simulink model "BuildingHeatLoadCalc"  (R2026a)
settings: Solver=ode1be  StopTime=31532400  FixedStep=3600  AbsTol=1e-3
undefined symbols (not defined in the file): BuildingThermalLib, lib_BuildingThermal
libraries: ExternalWall_lib x47, WallSelector_lib x36, fl_lib x32, RoomWithAirVolume x15, nesl_utility x4, TemperatureSource_lib x1, DayScheduler_lib x1, SolarRadiationAtLocation_lib x1
(part 2 of 5)

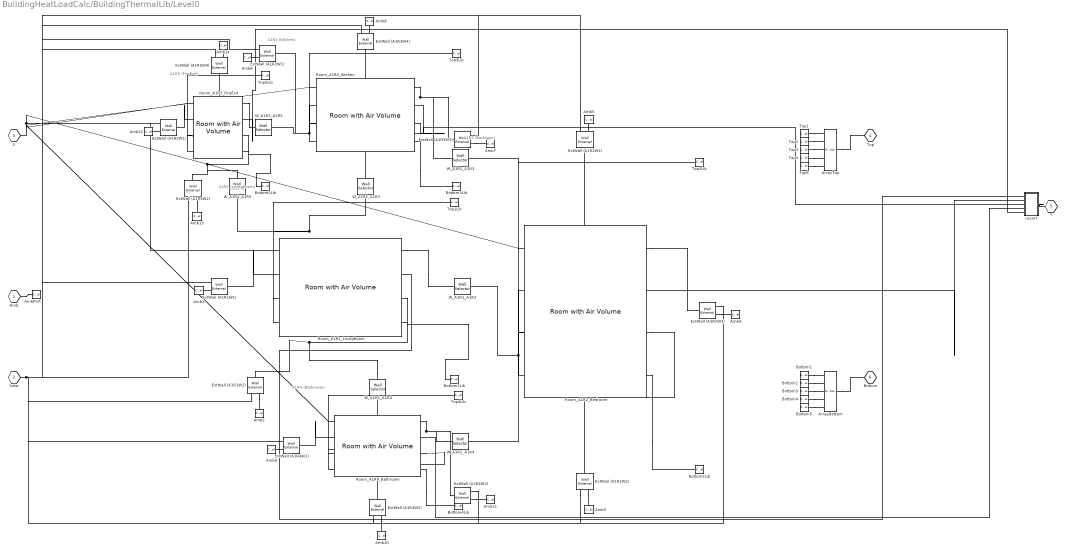
== system BuildingHeatLoadCalc/BuildingThermalLib/Level0 ==
  note: A1R1 (LivingRoom)
  note: A1R2 (Bedroom)
  note: A1R3 (Kitchen)
  note: A1R4 (Bathroom)
  note: A1R5 (FireExit)
  Amb{1..14} (14 alike) : ConnectionLabel  Label=A
  AmbPort : ConnectionLabel  Label=A
  ArrayBottom : SimscapeArrayConnection  Domain=foundation.thermal.thermal  ConcatenateDimension=1  NumScalarElements=5
  ArrayTop : SimscapeArrayConnection  Domain=foundation.thermal.thermal  ConcatenateDimension=1  NumScalarElements=5
  Bottom1 : ConnectionLabel  Label=Bottom1
  Bottom1Lib : ConnectionLabel  Label=Bottom1
  Bottom2 : ConnectionLabel  Label=Bottom2
  Bottom2Lib : ConnectionLabel  Label=Bottom2
  Bottom3 : ConnectionLabel  Label=Bottom3
  Bottom3Lib : ConnectionLabel  Label=Bottom3
  Bottom4 : ConnectionLabel  Label=Bottom4
  Bottom4Lib : ConnectionLabel  Label=Bottom4
  Bottom5 : ConnectionLabel  Label=Bottom5
  Bottom5Lib : ConnectionLabel  Label=Bottom5
  ExtWall (A1R1W1) : ExternalWall_lib/Wall External  extWallModel=wallExternalModelOption.wallSolarWin  wallLength=2.4384 % Parameterized on : 09-Jun-2026 19:35:12 m  wallHeight=3.048 % Parameterized on : 09-Jun-2026 19:35:12 m  wallThickness=0.07 % Parameterized on : 09-Jun-2026 19:35:12 m  wallMaterialDen=2000 % Parameterized on : 09-Jun-2026 19:35:13 kg/m^3  wallMaterialCp=1100 % Parameterized on : 09-Jun-2026 19:35:13 J/(K*kg)  wallAbsorptivity=0.6 % Parameterized on : 09-Jun-2026 19:35:13  wallThermalK=1.4 % Parameterized on : 09-Jun-2026 19:35:13 W/(K*m)  winLength=2.0401 % Parameterized on : 09-Jun-2026 19:35:12 m  winHeight=2.5501 % Parameterized on : 09-Jun-2026 19:35:12 m  winThickness=0.005 % Parameterized on : 09-Jun-2026 19:35:13 m  winMaterialDen=4000 % Parameterized on : 09-Jun-2026 19:35:13 kg/m^3  winMaterialCp=840 % Parameterized on : 09-Jun-2026 19:35:13 J/(K*kg)  winAbsorptivity=0.4 % Parameterized on : 09-Jun-2026 19:35:13  winThermalK=1 % Parameterized on : 09-Jun-2026 19:35:13 W/(K*m)  winTransmissivity=0.2 % Parameterized on : 09-Jun-2026 19:35:13  ventLength=0.1 m  ventHeight=0.1 m  extToWallHTC=20 % Parameterized on : 09-Jun-2026 19:35:13 W/(K*m^2)  intToRoomHTC=30 % Parameterized on : 09-Jun-2026 19:35:13 W/(K*m^2)  iniT=275.8 % Parameterized on : 09-Jun-2026 19:38:28 K  latitude=47.376 % Parameterized on : 09-Jun-2026 19:38:29  longitude=8.541 % Parameterized on : 09-Jun-2026 19:38:29  localTime=15.00 % Parameterized on : 09-Jun-2026 19:38:29  dayLightS=0 % Parameterized on : 09-Jun-2026 19:38:29  surfAngle=90 % Parameterized on : 09-Jun-2026 19:35:12 deg  surfUnitV="[-0.96593    -0.25882] % Parameterized on : 09-Jun-2026 19:35:12"  startYear=2024 % Parameterized on : 09-Jun-2026 19:38:29  startMonth=1 % Parameterized on : 09-Jun-2026 19:38:29  startDay=1 % Parameterized on : 09-Jun-2026 19:38:29  startHr=1 % Parameterized on : 09-Jun-2026 19:38:29  numHrsData=8760 % Parameterized on : 09-Jun-2026 19:38:29  interp_method=simscape.enum.interpolation.linear  extrap_method=simscape.enum.extrapolation.nearest
  ExtWall (A1R1W2) : ExternalWall_lib/Wall External  extWallModel=wallExternalModelOption.wallSolarWin  wallLength=3.048 % Parameterized on : 09-Jun-2026 19:35:12 m  wallHeight=3.048 % Parameterized on : 09-Jun-2026 19:35:12 m  wallThickness=0.07 % Parameterized on : 09-Jun-2026 19:35:12 m  wallMaterialDen=2000 % Parameterized on : 09-Jun-2026 19:35:13 kg/m^3  wallMaterialCp=1100 % Parameterized on : 09-Jun-2026 19:35:13 J/(K*kg)  wallAbsorptivity=0.6 % Parameterized on : 09-Jun-2026 19:35:13  wallThermalK=1.4 % Parameterized on : 09-Jun-2026 19:35:13 W/(K*m)  winLength=2.1552 % Parameterized on : 09-Jun-2026 19:35:12 m  winHeight=2.1553 % Parameterized on : 09-Jun-2026 19:35:12 m  winThickness=0.005 % Parameterized on : 09-Jun-2026 19:35:13 m  winMaterialDen=4000 % Parameterized on : 09-Jun-2026 19:35:13 kg/m^3  winMaterialCp=840 % Parameterized on : 09-Jun-2026 19:35:13 J/(K*kg)  winAbsorptivity=0.4 % Parameterized on : 09-Jun-2026 19:35:13  winThermalK=1 % Parameterized on : 09-Jun-2026 19:35:13 W/(K*m)  winTransmissivity=0.2 % Parameterized on : 09-Jun-2026 19:35:13  ventLength=0.1 m  ventHeight=0.1 m  extToWallHTC=20 % Parameterized on : 09-Jun-2026 19:35:13 W/(K*m^2)  intToRoomHTC=30 % Parameterized on : 09-Jun-2026 19:35:13 W/(K*m^2)  iniT=275.8 % Parameterized on : 09-Jun-2026 19:38:28 K  latitude=47.376 % Parameterized on : 09-Jun-2026 19:38:29  longitude=8.541 % Parameterized on : 09-Jun-2026 19:38:29  localTime=15.00 % Parameterized on : 09-Jun-2026 19:38:29  dayLightS=0 % Parameterized on : 09-Jun-2026 19:38:29  surfAngle=90 % Parameterized on : 09-Jun-2026 19:35:12 deg  surfUnitV="[-0.25882     0.96593] % Parameterized on : 09-Jun-2026 19:35:12"  startYear=2024 % Parameterized on : 09-Jun-2026 19:38:29  startMonth=1 % Parameterized on : 09-Jun-2026 19:38:29  startDay=1 % Parameterized on : 09-Jun-2026 19:38:29  startHr=1 % Parameterized on : 09-Jun-2026 19:38:29  numHrsData=8760 % Parameterized on : 09-Jun-2026 19:38:29  interp_method=simscape.enum.interpolation.linear  extrap_method=simscape.enum.extrapolation.nearest
  ExtWall (A1R2W2) : ExternalWall_lib/Wall External  extWallModel=wallExternalModelOption.wallSolar  wallLength=3.048 % Parameterized on : 09-Jun-2026 19:35:12 m  wallHeight=3.048 % Parameterized on : 09-Jun-2026 19:35:12 m  wallThickness=0.07 % Parameterized on : 09-Jun-2026 19:35:12 m  wallMaterialDen=2000 % Parameterized on : 09-Jun-2026 19:35:13 kg/m^3  wallMaterialCp=1100 % Parameterized on : 09-Jun-2026 19:35:13 J/(K*kg)  wallAbsorptivity=0.6 % Parameterized on : 09-Jun-2026 19:35:13  wallThermalK=1.4 % Parameterized on : 09-Jun-2026 19:35:13 W/(K*m)  winLength=1 m  winHeight=0.5 m  winThickness=0.007 m  winMaterialDen=2500 kg/m^3  winMaterialCp=787 J/(K*kg)  winAbsorptivity=0.35  winThermalK=1 W/(K*m)  winTransmissivity=0.45  ventLength=0.1 m  ventHeight=0.1 m  extToWallHTC=20 % Parameterized on : 09-Jun-2026 19:35:13 W/(K*m^2)  intToRoomHTC=30 % Parameterized on : 09-Jun-2026 19:35:13 W/(K*m^2)  iniT=275.8 % Parameterized on : 09-Jun-2026 19:38:28 K  latitude=47.376 % Parameterized on : 09-Jun-2026 19:38:29  longitude=8.541 % Parameterized on : 09-Jun-2026 19:38:29  localTime=15.00 % Parameterized on : 09-Jun-2026 19:38:29  dayLightS=0 % Parameterized on : 09-Jun-2026 19:38:29  surfAngle=90 % Parameterized on : 09-Jun-2026 19:35:12 deg  surfUnitV="[-0.25882     0.96593] % Parameterized on : 09-Jun-2026 19:35:12"  startYear=2024 % Parameterized on : 09-Jun-2026 19:38:29  startMonth=1 % Parameterized on : 09-Jun-2026 19:38:29  startDay=1 % Parameterized on : 09-Jun-2026 19:38:29  startHr=1 % Parameterized on : 09-Jun-2026 19:38:29  numHrsData=8760 % Parameterized on : 09-Jun-2026 19:38:29  interp_method=simscape.enum.interpolation.linear  extrap_method=simscape.enum.extrapolation.nearest
  ExtWall (A1R2W3) : ExternalWall_lib/Wall External  extWallModel=wallExternalModelOption.wallSolarWin  wallLength=4.2672 % Parameterized on : 09-Jun-2026 19:35:12 m  wallHeight=3.048 % Parameterized on : 09-Jun-2026 19:35:12 m  wallThickness=0.07 % Parameterized on : 09-Jun-2026 19:35:12 m  wallMaterialDen=2000 % Parameterized on : 09-Jun-2026 19:35:13 kg/m^3  wallMaterialCp=1100 % Parameterized on : 09-Jun-2026 19:35:13 J/(K*kg)  wallAbsorptivity=0.6 % Parameterized on : 09-Jun-2026 19:35:13  wallThermalK=1.4 % Parameterized on : 09-Jun-2026 19:35:13 W/(K*m)  winLength=3.5702 % Parameterized on : 09-Jun-2026 19:35:12 m  winHeight=2.5501 % Parameterized on : 09-Jun-2026 19:35:12 m  winThickness=0.005 % Parameterized on : 09-Jun-2026 19:35:13 m  winMaterialDen=4000 % Parameterized on : 09-Jun-2026 19:35:13 kg/m^3  winMaterialCp=840 % Parameterized on : 09-Jun-2026 19:35:13 J/(K*kg)  winAbsorptivity=0.4 % Parameterized on : 09-Jun-2026 19:35:13  winThermalK=1 % Parameterized on : 09-Jun-2026 19:35:13 W/(K*m)  winTransmissivity=0.2 % Parameterized on : 09-Jun-2026 19:35:13  ventLength=0.1 m  ventHeight=0.1 m  extToWallHTC=20 % Parameterized on : 09-Jun-2026 19:35:13 W/(K*m^2)  intToRoomHTC=30 % Parameterized on : 09-Jun-2026 19:35:13 W/(K*m^2)  iniT=275.8 % Parameterized on : 09-Jun-2026 19:38:28 K  latitude=47.376 % Parameterized on : 09-Jun-2026 19:38:29  longitude=8.541 % Parameterized on : 09-Jun-2026 19:38:29  localTime=15.00 % Parameterized on : 09-Jun-2026 19:38:29  dayLightS=0 % Parameterized on : 09-Jun-2026 19:38:29  surfAngle=90 % Parameterized on : 09-Jun-2026 19:35:12 deg  surfUnitV="[0.96593     0.25882] % Parameterized on : 09-Jun-2026 19:35:12"  startYear=2024 % Parameterized on : 09-Jun-2026 19:38:29  startMonth=1 % Parameterized on : 09-Jun-2026 19:38:29  startDay=1 % Parameterized on : 09-Jun-2026 19:38:29  startHr=1 % Parameterized on : 09-Jun-2026 19:38:29  numHrsData=8760 % Parameterized on : 09-Jun-2026 19:38:29  interp_method=simscape.enum.interpolation.linear  extrap_method=simscape.enum.extrapolation.nearest
  ExtWall (A1R2W4) : ExternalWall_lib/Wall External  extWallModel=wallExternalModelOption.wallSolarWin  wallLength=3.048 % Parameterized on : 09-Jun-2026 19:35:12 m  wallHeight=3.048 % Parameterized on : 09-Jun-2026 19:35:12 m  wallThickness=0.07 % Parameterized on : 09-Jun-2026 19:35:12 m  wallMaterialDen=2000 % Parameterized on : 09-Jun-2026 19:35:13 kg/m^3  wallMaterialCp=1100 % Parameterized on : 09-Jun-2026 19:35:13 J/(K*kg)  wallAbsorptivity=0.6 % Parameterized on : 09-Jun-2026 19:35:13  wallThermalK=1.4 % Parameterized on : 09-Jun-2026 19:35:13 W/(K*m)  winLength=2.1552 % Parameterized on : 09-Jun-2026 19:35:12 m  winHeight=2.1553 % Parameterized on : 09-Jun-2026 19:35:12 m  winThickness=0.005 % Parameterized on : 09-Jun-2026 19:35:13 m  winMaterialDen=4000 % Parameterized on : 09-Jun-2026 19:35:13 kg/m^3  winMaterialCp=840 % Parameterized on : 09-Jun-2026 19:35:13 J/(K*kg)  winAbsorptivity=0.4 % Parameterized on : 09-Jun-2026 19:35:13  winThermalK=1 % Parameterized on : 09-Jun-2026 19:35:13 W/(K*m)  winTransmissivity=0.2 % Parameterized on : 09-Jun-2026 19:35:13  ventLength=0.1 m  ventHeight=0.1 m  extToWallHTC=20 % Parameterized on : 09-Jun-2026 19:35:13 W/(K*m^2)  intToRoomHTC=30 % Parameterized on : 09-Jun-2026 19:35:13 W/(K*m^2)  iniT=275.8 % Parameterized on : 09-Jun-2026 19:38:28 K  latitude=47.376 % Parameterized on : 09-Jun-2026 19:38:29  longitude=8.541 % Parameterized on : 09-Jun-2026 19:38:29  localTime=15.00 % Parameterized on : 09-Jun-2026 19:38:29  dayLightS=0 % Parameterized on : 09-Jun-2026 19:38:29  surfAngle=90 % Parameterized on : 09-Jun-2026 19:35:12 deg  surfUnitV="[0.25882    -0.96593] % Parameterized on : 09-Jun-2026 19:35:12"  startYear=2024 % Parameterized on : 09-Jun-2026 19:38:29  startMonth=1 % Parameterized on : 09-Jun-2026 19:38:29  startDay=1 % Parameterized on : 09-Jun-2026 19:38:29  startHr=1 % Parameterized on : 09-Jun-2026 19:38:29  numHrsData=8760 % Parameterized on : 09-Jun-2026 19:38:29  interp_method=simscape.enum.interpolation.linear  extrap_method=simscape.enum.extrapolation.nearest
  ExtWall (A1R3W1) : ExternalWall_lib/Wall External  extWallModel=wallExternalModelOption.wallSolar  wallLength=1.8288 % Parameterized on : 09-Jun-2026 19:35:12 m  wallHeight=3.048 % Parameterized on : 09-Jun-2026 19:35:12 m  wallThickness=0.07 % Parameterized on : 09-Jun-2026 19:35:12 m  wallMaterialDen=2000 % Parameterized on : 09-Jun-2026 19:35:13 kg/m^3  wallMaterialCp=1100 % Parameterized on : 09-Jun-2026 19:35:13 J/(K*kg)  wallAbsorptivity=0.6 % Parameterized on : 09-Jun-2026 19:35:13  wallThermalK=1.4 % Parameterized on : 09-Jun-2026 19:35:13 W/(K*m)  winLength=1 m  winHeight=0.5 m  winThickness=0.007 m  winMaterialDen=2500 kg/m^3  winMaterialCp=787 J/(K*kg)  winAbsorptivity=0.35  winThermalK=1 W/(K*m)  winTransmissivity=0.45  ventLength=0.1 m  ventHeight=0.1 m  extToWallHTC=20 % Parameterized on : 09-Jun-2026 19:35:13 W/(K*m^2)  intToRoomHTC=30 % Parameterized on : 09-Jun-2026 19:35:13 W/(K*m^2)  iniT=275.8 % Parameterized on : 09-Jun-2026 19:38:28 K  latitude=47.376 % Parameterized on : 09-Jun-2026 19:38:29  longitude=8.541 % Parameterized on : 09-Jun-2026 19:38:29  localTime=15.00 % Parameterized on : 09-Jun-2026 19:38:29  dayLightS=0 % Parameterized on : 09-Jun-2026 19:38:29  surfAngle=90 % Parameterized on : 09-Jun-2026 19:35:12 deg  surfUnitV="[-0.96593    -0.25882] % Parameterized on : 09-Jun-2026 19:35:12"  startYear=2024 % Parameterized on : 09-Jun-2026 19:38:29  startMonth=1 % Parameterized on : 09-Jun-2026 19:38:29  startDay=1 % Parameterized on : 09-Jun-2026 19:38:29  startHr=1 % Parameterized on : 09-Jun-2026 19:38:29  numHrsData=8760 % Parameterized on : 09-Jun-2026 19:38:29  interp_method=simscape.enum.interpolation.linear  extrap_method=simscape.enum.extrapolation.nearest
  ExtWall (A1R3W3) : ExternalWall_lib/Wall External  extWallModel=wallExternalModelOption.wallSolarWin  wallLength=1.8289 % Parameterized on : 09-Jun-2026 19:35:12 m  wallHeight=3.048 % Parameterized on : 09-Jun-2026 19:35:12 m  wallThickness=0.07 % Parameterized on : 09-Jun-2026 19:35:12 m  wallMaterialDen=2000 % Parameterized on : 09-Jun-2026 19:35:13 kg/m^3  wallMaterialCp=1100 % Parameterized on : 09-Jun-2026 19:35:13 J/(K*kg)  wallAbsorptivity=0.6 % Parameterized on : 09-Jun-2026 19:35:13  wallThermalK=1.4 % Parameterized on : 09-Jun-2026 19:35:13 W/(K*m)  winLength=1.5301 % Parameterized on : 09-Jun-2026 19:35:12 m  winHeight=2.5501 % Parameterized on : 09-Jun-2026 19:35:12 m  winThickness=0.005 % Parameterized on : 09-Jun-2026 19:35:13 m  winMaterialDen=4000 % Parameterized on : 09-Jun-2026 19:35:13 kg/m^3  winMaterialCp=840 % Parameterized on : 09-Jun-2026 19:35:13 J/(K*kg)  winAbsorptivity=0.4 % Parameterized on : 09-Jun-2026 19:35:13  winThermalK=1 % Parameterized on : 09-Jun-2026 19:35:13 W/(K*m)  winTransmissivity=0.2 % Parameterized on : 09-Jun-2026 19:35:13  ventLength=0.1 m  ventHeight=0.1 m  extToWallHTC=20 % Parameterized on : 09-Jun-2026 19:35:13 W/(K*m^2)  intToRoomHTC=30 % Parameterized on : 09-Jun-2026 19:35:13 W/(K*m^2)  iniT=275.8 % Parameterized on : 09-Jun-2026 19:38:28 K  latitude=47.376 % Parameterized on : 09-Jun-2026 19:38:29  longitude=8.541 % Parameterized on : 09-Jun-2026 19:38:29  localTime=15.00 % Parameterized on : 09-Jun-2026 19:38:29  dayLightS=0 % Parameterized on : 09-Jun-2026 19:38:29  surfAngle=90 % Parameterized on : 09-Jun-2026 19:35:12 deg  surfUnitV="[0.96593     0.25882] % Parameterized on : 09-Jun-2026 19:35:12"  startYear=2024 % Parameterized on : 09-Jun-2026 19:38:29  startMonth=1 % Parameterized on : 09-Jun-2026 19:38:29  startDay=1 % Parameterized on : 09-Jun-2026 19:38:29  startHr=1 % Parameterized on : 09-Jun-2026 19:38:29  numHrsData=8760 % Parameterized on : 09-Jun-2026 19:38:29  interp_method=simscape.enum.interpolation.linear  extrap_method=simscape.enum.extrapolation.nearest
  ExtWall (A1R3W4) : ExternalWall_lib/Wall External  extWallModel=wallExternalModelOption.wallSolarWin  wallLength=2.4385 % Parameterized on : 09-Jun-2026 19:35:12 m  wallHeight=3.048 % Parameterized on : 09-Jun-2026 19:35:12 m  wallThickness=0.07 % Parameterized on : 09-Jun-2026 19:35:12 m  wallMaterialDen=2000 % Parameterized on : 09-Jun-2026 19:35:13 kg/m^3  wallMaterialCp=1100 % Parameterized on : 09-Jun-2026 19:35:13 J/(K*kg)  wallAbsorptivity=0.6 % Parameterized on : 09-Jun-2026 19:35:13  wallThermalK=1.4 % Parameterized on : 09-Jun-2026 19:35:13 W/(K*m)  winLength=2.0402 % Parameterized on : 09-Jun-2026 19:35:12 m  winHeight=2.5501 % Parameterized on : 09-Jun-2026 19:35:12 m  winThickness=0.005 % Parameterized on : 09-Jun-2026 19:35:13 m  winMaterialDen=4000 % Parameterized on : 09-Jun-2026 19:35:13 kg/m^3  winMaterialCp=840 % Parameterized on : 09-Jun-2026 19:35:13 J/(K*kg)  winAbsorptivity=0.4 % Parameterized on : 09-Jun-2026 19:35:13  winThermalK=1 % Parameterized on : 09-Jun-2026 19:35:13 W/(K*m)  winTransmissivity=0.2 % Parameterized on : 09-Jun-2026 19:35:13  ventLength=0.1 m  ventHeight=0.1 m  extToWallHTC=20 % Parameterized on : 09-Jun-2026 19:35:13 W/(K*m^2)  intToRoomHTC=30 % Parameterized on : 09-Jun-2026 19:35:13 W/(K*m^2)  iniT=275.8 % Parameterized on : 09-Jun-2026 19:38:28 K  latitude=47.376 % Parameterized on : 09-Jun-2026 19:38:29  longitude=8.541 % Parameterized on : 09-Jun-2026 19:38:29  localTime=15.00 % Parameterized on : 09-Jun-2026 19:38:29  dayLightS=0 % Parameterized on : 09-Jun-2026 19:38:29  surfAngle=90 % Parameterized on : 09-Jun-2026 19:35:12 deg  surfUnitV="[0.25882    -0.96593] % Parameterized on : 09-Jun-2026 19:35:12"  startYear=2024 % Parameterized on : 09-Jun-2026 19:38:29  startMonth=1 % Parameterized on : 09-Jun-2026 19:38:29  startDay=1 % Parameterized on : 09-Jun-2026 19:38:29  startHr=1 % Parameterized on : 09-Jun-2026 19:38:29  numHrsData=8760 % Parameterized on : 09-Jun-2026 19:38:29  interp_method=simscape.enum.interpolation.linear  extrap_method=simscape.enum.extrapolation.nearest
  ExtWall (A1R4W1) : ExternalWall_lib/Wall External  extWallModel=wallExternalModelOption.wallSolar  wallLength=1.524 % Parameterized on : 09-Jun-2026 19:35:12 m  wallHeight=3.048 % Parameterized on : 09-Jun-2026 19:35:12 m  wallThickness=0.07 % Parameterized on : 09-Jun-2026 19:35:12 m  wallMaterialDen=2000 % Parameterized on : 09-Jun-2026 19:35:13 kg/m^3  wallMaterialCp=1100 % Parameterized on : 09-Jun-2026 19:35:13 J/(K*kg)  wallAbsorptivity=0.6 % Parameterized on : 09-Jun-2026 19:35:13  wallThermalK=1.4 % Parameterized on : 09-Jun-2026 19:35:13 W/(K*m)  winLength=1 m  winHeight=0.5 m  winThickness=0.007 m  winMaterialDen=2500 kg/m^3  winMaterialCp=787 J/(K*kg)  winAbsorptivity=0.35  winThermalK=1 W/(K*m)  winTransmissivity=0.45  ventLength=0.1 m  ventHeight=0.1 m  extToWallHTC=20 % Parameterized on : 09-Jun-2026 19:35:13 W/(K*m^2)  intToRoomHTC=30 % Parameterized on : 09-Jun-2026 19:35:13 W/(K*m^2)  iniT=275.8 % Parameterized on : 09-Jun-2026 19:38:28 K  latitude=47.376 % Parameterized on : 09-Jun-2026 19:38:29  longitude=8.541 % Parameterized on : 09-Jun-2026 19:38:29  localTime=15.00 % Parameterized on : 09-Jun-2026 19:38:29  dayLightS=0 % Parameterized on : 09-Jun-2026 19:38:29  surfAngle=90 % Parameterized on : 09-Jun-2026 19:35:12 deg  surfUnitV="[-0.96593    -0.25882] % Parameterized on : 09-Jun-2026 19:35:12"  startYear=2024 % Parameterized on : 09-Jun-2026 19:38:29  startMonth=1 % Parameterized on : 09-Jun-2026 19:38:29  startDay=1 % Parameterized on : 09-Jun-2026 19:38:29  startHr=1 % Parameterized on : 09-Jun-2026 19:38:29  numHrsData=8760 % Parameterized on : 09-Jun-2026 19:38:29  interp_method=simscape.enum.interpolation.linear  extrap_method=simscape.enum.extrapolation.nearest
  ExtWall (A1R4W2) : ExternalWall_lib/Wall External  extWallModel=wallExternalModelOption.wallSolarWin  wallLength=2.1336 % Parameterized on : 09-Jun-2026 19:35:12 m  wallHeight=3.048 % Parameterized on : 09-Jun-2026 19:35:12 m  wallThickness=0.07 % Parameterized on : 09-Jun-2026 19:35:12 m  wallMaterialDen=2000 % Parameterized on : 09-Jun-2026 19:35:13 kg/m^3  wallMaterialCp=1100 % Parameterized on : 09-Jun-2026 19:35:14 J/(K*kg)  wallAbsorptivity=0.6 % Parameterized on : 09-Jun-2026 19:35:14  wallThermalK=1.4 % Parameterized on : 09-Jun-2026 19:35:14 W/(K*m)  winLength=1.1686 % Parameterized on : 09-Jun-2026 19:35:12 m  winHeight=1.6695 % Parameterized on : 09-Jun-2026 19:35:12 m  winThickness=0.005 % Parameterized on : 09-Jun-2026 19:35:14 m  winMaterialDen=4000 % Parameterized on : 09-Jun-2026 19:35:14 kg/m^3  winMaterialCp=840 % Parameterized on : 09-Jun-2026 19:35:14 J/(K*kg)  winAbsorptivity=0.4 % Parameterized on : 09-Jun-2026 19:35:14  winThermalK=1 % Parameterized on : 09-Jun-2026 19:35:14 W/(K*m)  winTransmissivity=0.2 % Parameterized on : 09-Jun-2026 19:35:14  ventLength=0.1 m  ventHeight=0.1 m  extToWallHTC=20 % Parameterized on : 09-Jun-2026 19:35:14 W/(K*m^2)  intToRoomHTC=30 % Parameterized on : 09-Jun-2026 19:35:14 W/(K*m^2)  iniT=275.8 % Parameterized on : 09-Jun-2026 19:38:28 K  latitude=47.376 % Parameterized on : 09-Jun-2026 19:38:29  longitude=8.541 % Parameterized on : 09-Jun-2026 19:38:29  localTime=15.00 % Parameterized on : 09-Jun-2026 19:38:29  dayLightS=0 % Parameterized on : 09-Jun-2026 19:38:29  surfAngle=90 % Parameterized on : 09-Jun-2026 19:35:12 deg  surfUnitV="[-0.25882     0.96593] % Parameterized on : 09-Jun-2026 19:35:12"  startYear=2024 % Parameterized on : 09-Jun-2026 19:38:29  startMonth=1 % Parameterized on : 09-Jun-2026 19:38:29  startDay=1 % Parameterized on : 09-Jun-2026 19:38:29  startHr=1 % Parameterized on : 09-Jun-2026 19:38:29  numHrsData=8760 % Parameterized on : 09-Jun-2026 19:38:29  interp_method=simscape.enum.interpolation.linear  extrap_method=simscape.enum.extrapolation.nearest
  ExtWall (A1R4W3) : ExternalWall_lib/Wall External  extWallModel=wallExternalModelOption.wallSolar  wallLength=1.524 % Parameterized on : 09-Jun-2026 19:35:12 m  wallHeight=3.048 % Parameterized on : 09-Jun-2026 19:35:12 m  wallThickness=0.07 % Parameterized on : 09-Jun-2026 19:35:12 m  wallMaterialDen=2000 % Parameterized on : 09-Jun-2026 19:35:14 kg/m^3  wallMaterialCp=1100 % Parameterized on : 09-Jun-2026 19:35:14 J/(K*kg)  wallAbsorptivity=0.6 % Parameterized on : 09-Jun-2026 19:35:14  wallThermalK=1.4 % Parameterized on : 09-Jun-2026 19:35:14 W/(K*m)  winLength=1 m  winHeight=0.5 m  winThickness=0.007 m  winMaterialDen=2500 kg/m^3  winMaterialCp=787 J/(K*kg)  winAbsorptivity=0.35  winThermalK=1 W/(K*m)  winTransmissivity=0.45  ventLength=0.1 m  ventHeight=0.1 m  extToWallHTC=20 % Parameterized on : 09-Jun-2026 19:35:14 W/(K*m^2)  intToRoomHTC=30 % Parameterized on : 09-Jun-2026 19:35:14 W/(K*m^2)  iniT=275.8 % Parameterized on : 09-Jun-2026 19:38:28 K  latitude=47.376 % Parameterized on : 09-Jun-2026 19:38:29  longitude=8.541 % Parameterized on : 09-Jun-2026 19:38:29  localTime=15.00 % Parameterized on : 09-Jun-2026 19:38:29  dayLightS=0 % Parameterized on : 09-Jun-2026 19:38:29  surfAngle=90 % Parameterized on : 09-Jun-2026 19:35:12 deg  surfUnitV="[0.96593     0.25882] % Parameterized on : 09-Jun-2026 19:35:12"  startYear=2024 % Parameterized on : 09-Jun-2026 19:38:29  startMonth=1 % Parameterized on : 09-Jun-2026 19:38:29  startDay=1 % Parameterized on : 09-Jun-2026 19:38:29  startHr=1 % Parameterized on : 09-Jun-2026 19:38:29  numHrsData=8760 % Parameterized on : 09-Jun-2026 19:38:29  interp_method=simscape.enum.interpolation.linear  extrap_method=simscape.enum.extrapolation.nearest
  ExtWall (A1R5W1) : ExternalWall_lib/Wall External  extWallModel=wallExternalModelOption.wallSolar  wallLength=1.524 % Parameterized on : 09-Jun-2026 19:35:12 m  wallHeight=3.048 % Parameterized on : 09-Jun-2026 19:35:12 m  wallThickness=0.07 % Parameterized on : 09-Jun-2026 19:35:12 m  wallMaterialDen=2000 % Parameterized on : 09-Jun-2026 19:35:14 kg/m^3  wallMaterialCp=1100 % Parameterized on : 09-Jun-2026 19:35:14 J/(K*kg)  wallAbsorptivity=0.6 % Parameterized on : 09-Jun-2026 19:35:14  wallThermalK=1.4 % Parameterized on : 09-Jun-2026 19:35:14 W/(K*m)  winLength=1 m  winHeight=0.5 m  winThickness=0.007 m  winMaterialDen=2500 kg/m^3  winMaterialCp=787 J/(K*kg)  winAbsorptivity=0.35  winThermalK=1 W/(K*m)  winTransmissivity=0.45  ventLength=0.1 m  ventHeight=0.1 m  extToWallHTC=20 % Parameterized on : 09-Jun-2026 19:35:14 W/(K*m^2)  intToRoomHTC=30 % Parameterized on : 09-Jun-2026 19:35:14 W/(K*m^2)  iniT=275.8 % Parameterized on : 09-Jun-2026 19:38:28 K  latitude=47.376 % Parameterized on : 09-Jun-2026 19:38:29  longitude=8.541 % Parameterized on : 09-Jun-2026 19:38:29  localTime=15.00 % Parameterized on : 09-Jun-2026 19:38:29  dayLightS=0 % Parameterized on : 09-Jun-2026 19:38:29  surfAngle=90 % Parameterized on : 09-Jun-2026 19:35:12 deg  surfUnitV="[-0.96593    -0.25882] % Parameterized on : 09-Jun-2026 19:35:12"  startYear=2024 % Parameterized on : 09-Jun-2026 19:38:29  startMonth=1 % Parameterized on : 09-Jun-2026 19:38:29  startDay=1 % Parameterized on : 09-Jun-2026 19:38:29  startHr=1 % Parameterized on : 09-Jun-2026 19:38:29  numHrsData=8760 % Parameterized on : 09-Jun-2026 19:38:29  interp_method=simscape.enum.interpolation.linear  extrap_method=simscape.enum.extrapolation.nearest
  ExtWall (A1R5W2) : ExternalWall_lib/Wall External  extWallModel=wallExternalModelOption.wallSolar  wallLength=1.2192 % Parameterized on : 09-Jun-2026 19:35:12 m  wallHeight=3.048 % Parameterized on : 09-Jun-2026 19:35:12 m  wallThickness=0.07 % Parameterized on : 09-Jun-2026 19:35:12 m  wallMaterialDen=2000 % Parameterized on : 09-Jun-2026 19:35:14 kg/m^3  wallMaterialCp=1100 % Parameterized on : 09-Jun-2026 19:35:14 J/(K*kg)  wallAbsorptivity=0.6 % Parameterized on : 09-Jun-2026 19:35:14  wallThermalK=1.4 % Parameterized on : 09-Jun-2026 19:35:14 W/(K*m)  winLength=1 m  winHeight=0.5 m  winThickness=0.007 m  winMaterialDen=2500 kg/m^3  winMaterialCp=787 J/(K*kg)  winAbsorptivity=0.35  winThermalK=1 W/(K*m)  winTransmissivity=0.45  ventLength=0.1 m  ventHeight=0.1 m  extToWallHTC=20 % Parameterized on : 09-Jun-2026 19:35:14 W/(K*m^2)  intToRoomHTC=30 % Parameterized on : 09-Jun-2026 19:35:14 W/(K*m^2)  iniT=275.8 % Parameterized on : 09-Jun-2026 19:38:28 K  latitude=47.376 % Parameterized on : 09-Jun-2026 19:38:29  longitude=8.541 % Parameterized on : 09-Jun-2026 19:38:29  localTime=15.00 % Parameterized on : 09-Jun-2026 19:38:29  dayLightS=0 % Parameterized on : 09-Jun-2026 19:38:29  surfAngle=90 % Parameterized on : 09-Jun-2026 19:35:12 deg  surfUnitV="[-0.25882     0.96593] % Parameterized on : 09-Jun-2026 19:35:12"  startYear=2024 % Parameterized on : 09-Jun-2026 19:38:29  startMonth=1 % Parameterized on : 09-Jun-2026 19:38:29  startDay=1 % Parameterized on : 09-Jun-2026 19:38:29  startHr=1 % Parameterized on : 09-Jun-2026 19:38:29  numHrsData=8760 % Parameterized on : 09-Jun-2026 19:38:29  interp_method=simscape.enum.interpolation.linear  extrap_method=simscape.enum.extrapolation.nearest
  ExtWall (A1R5W4) : ExternalWall_lib/Wall External  extWallModel=wallExternalModelOption.wallSolarWin  wallLength=1.2192 % Parameterized on : 09-Jun-2026 19:35:12 m  wallHeight=3.048 % Parameterized on : 09-Jun-2026 19:35:12 m  wallThickness=0.07 % Parameterized on : 09-Jun-2026 19:35:12 m  wallMaterialDen=2000 % Parameterized on : 09-Jun-2026 19:35:14 kg/m^3  wallMaterialCp=1100 % Parameterized on : 09-Jun-2026 19:35:14 J/(K*kg)  wallAbsorptivity=0.6 % Parameterized on : 09-Jun-2026 19:35:14  wallThermalK=1.4 % Parameterized on : 09-Jun-2026 19:35:14 W/(K*m)  winLength=0.9444 % Parameterized on : 09-Jun-2026 19:35:12 m  winHeight=2.361 % Parameterized on : 09-Jun-2026 19:35:12 m  winThickness=0.005 % Parameterized on : 09-Jun-2026 19:35:14 m  winMaterialDen=4000 % Parameterized on : 09-Jun-2026 19:35:14 kg/m^3  winMaterialCp=840 % Parameterized on : 09-Jun-2026 19:35:14 J/(K*kg)  winAbsorptivity=0.4 % Parameterized on : 09-Jun-2026 19:35:14  winThermalK=1 % Parameterized on : 09-Jun-2026 19:35:14 W/(K*m)  winTransmissivity=0.2 % Parameterized on : 09-Jun-2026 19:35:14  ventLength=0.1 m  ventHeight=0.1 m  extToWallHTC=20 % Parameterized on : 09-Jun-2026 19:35:14 W/(K*m^2)  intToRoomHTC=30 % Parameterized on : 09-Jun-2026 19:35:14 W/(K*m^2)  iniT=275.8 % Parameterized on : 09-Jun-2026 19:38:28 K  latitude=47.376 % Parameterized on : 09-Jun-2026 19:38:29  longitude=8.541 % Parameterized on : 09-Jun-2026 19:38:29  localTime=15.00 % Parameterized on : 09-Jun-2026 19:38:29  dayLightS=0 % Parameterized on : 09-Jun-2026 19:38:29  surfAngle=90 % Parameterized on : 09-Jun-2026 19:35:12 deg  surfUnitV="[0.25882    -0.96593] % Parameterized on : 09-Jun-2026 19:35:12"  startYear=2024 % Parameterized on : 09-Jun-2026 19:38:29  startMonth=1 % Parameterized on : 09-Jun-2026 19:38:29  startDay=1 % Parameterized on : 09-Jun-2026 19:38:29  startHr=1 % Parameterized on : 09-Jun-2026 19:38:29  numHrsData=8760 % Parameterized on : 09-Jun-2026 19:38:29  interp_method=simscape.enum.interpolation.linear  extrap_method=simscape.enum.extrapolation.nearest
  Room_A1R1_LivingRoom : RoomWithAirVolume/Room with Air Volume  roomWid=3.048 % Parameterized on : 09-Jun-2026 19:35:12  roomHgt=3.048 % Parameterized on : 09-Jun-2026 19:35:12  roomLen=2.4384 % Parameterized on : 09-Jun-2026 19:35:12  htc=30 % Parameterized on : 09-Jun-2026 19:35:13  iniT=275.8 % Parameterized on : 09-Jun-2026 19:38:28  indxS=1
  Room_A1R2_Bedroom : RoomWithAirVolume/Room with Air Volume  roomWid=3.048 % Parameterized on : 09-Jun-2026 19:35:12  roomHgt=3.048 % Parameterized on : 09-Jun-2026 19:35:12  roomLen=4.2672 % Parameterized on : 09-Jun-2026 19:35:12  htc=30 % Parameterized on : 09-Jun-2026 19:35:13  iniT=275.8 % Parameterized on : 09-Jun-2026 19:38:28  indxS=2
  Room_A1R3_Kitchen : RoomWithAirVolume/Room with Air Volume  roomWid=2.4384 % Parameterized on : 09-Jun-2026 19:35:12  roomHgt=3.048 % Parameterized on : 09-Jun-2026 19:35:12  roomLen=1.8288 % Parameterized on : 09-Jun-2026 19:35:12  htc=30 % Parameterized on : 09-Jun-2026 19:35:13  iniT=275.8 % Parameterized on : 09-Jun-2026 19:38:28  indxS=3
  Room_A1R4_Bathroom : RoomWithAirVolume/Room with Air Volume  roomWid=2.1336 % Parameterized on : 09-Jun-2026 19:35:12  roomHgt=3.048 % Parameterized on : 09-Jun-2026 19:35:12  roomLen=1.524 % Parameterized on : 09-Jun-2026 19:35:12  htc=30 % Parameterized on : 09-Jun-2026 19:35:13  iniT=275.8 % Parameterized on : 09-Jun-2026 19:38:28  indxS=4
  Room_A1R5_FireExit : RoomWithAirVolume/Room with Air Volume  roomWid=1.2192 % Parameterized on : 09-Jun-2026 19:35:12  roomHgt=3.048 % Parameterized on : 09-Jun-2026 19:35:12  roomLen=1.524 % Parameterized on : 09-Jun-2026 19:35:12  htc=30 % Parameterized on : 09-Jun-2026 19:35:13  iniT=275.8 % Parameterized on : 09-Jun-2026 19:38:28  indxS=5
  Top1 : ConnectionLabel  Label=Top1
  Top1Lib : ConnectionLabel  Label=Top1
  Top2 : ConnectionLabel  Label=Top2
  Top2Lib : ConnectionLabel  Label=Top2
  Top3 : ConnectionLabel  Label=Top3
  Top3Lib : ConnectionLabel  Label=Top3
  Top4 : ConnectionLabel  Label=Top4
  Top4Lib : ConnectionLabel  Label=Top4
  Top5 : ConnectionLabel  Label=Top5
  Top5Lib : ConnectionLabel  Label=Top5
  W_A1R1_A1R2 : WallSelector_lib/Wall Selector  optWall=wallModelOption.wallWinVent  wallLength=2.4384 % Parameterized on : 09-Jun-2026 19:35:13 m  wallHeight=3.048 % Parameterized on : 09-Jun-2026 19:35:13 m  wallThickness=0.04 % Parameterized on : 09-Jun-2026 19:35:13 m  wallMaterialDen=650 % Parameterized on : 09-Jun-2026 19:35:15 kg/m^3  wallMaterialCp=1100 % Parameterized on : 09-Jun-2026 19:35:15 J/(K*kg)  wallAbsorptivity=0.5  wallThermalK=1.4 % Parameterized on : 09-Jun-2026 19:35:15 W/(K*m)  winLength=1 m  winHeight=0.5 m  winThickness=0.007 m  winMaterialDen=2500 kg/m^3  winMaterialCp=787 J/(K*kg)  winAbsorptivity=0.35  winThermalK=1 W/(K*m)  winTransmissivity=0.45  ventLength=1.2192 % Parameterized on : 09-Jun-2026 19:35:13 m  ventHeight=1.524 % Parameterized on : 09-Jun-2026 19:35:13 m  extToWallHTC=30 % Parameterized on : 09-Jun-2026 19:35:15 W/(K*m^2)  intToRoomHTC=30 % Parameterized on : 09-Jun-2026 19:35:15 W/(K*m^2)  iniT=275.8 % Parameterized on : 09-Jun-2026 19:38:28 K
  W_A1R1_A1R3 : WallSelector_lib/Wall Selector  optWall=wallModelOption.wallWinVent  wallLength=2.4383 % Parameterized on : 09-Jun-2026 19:35:13 m  wallHeight=3.048 % Parameterized on : 09-Jun-2026 19:35:13 m  wallThickness=0.04 % Parameterized on : 09-Jun-2026 19:35:13 m  wallMaterialDen=650 % Parameterized on : 09-Jun-2026 19:35:15 kg/m^3  wallMaterialCp=1100 % Parameterized on : 09-Jun-2026 19:35:15 J/(K*kg)  wallAbsorptivity=0.5  wallThermalK=1.4 % Parameterized on : 09-Jun-2026 19:35:15 W/(K*m)  winLength=1 m  winHeight=0.5 m  winThickness=0.007 m  winMaterialDen=2500 kg/m^3  winMaterialCp=787 J/(K*kg)  winAbsorptivity=0.35  winThermalK=1 W/(K*m)  winTransmissivity=0.45  ventLength=1.7242 % Parameterized on : 09-Jun-2026 19:35:13 m  ventHeight=2.1553 % Parameterized on : 09-Jun-2026 19:35:13 m  extToWallHTC=30 % Parameterized on : 09-Jun-2026 19:35:15 W/(K*m^2)  intToRoomHTC=30 % Parameterized on : 09-Jun-2026 19:35:15 W/(K*m^2)  iniT=275.8 % Parameterized on : 09-Jun-2026 19:38:28 K
  W_A1R1_A1R4 : WallSelector_lib/Wall Selector  optWall=wallModelOption.wallOnly  wallLength=2.1336 % Parameterized on : 09-Jun-2026 19:35:13 m  wallHeight=3.048 % Parameterized on : 09-Jun-2026 19:35:13 m  wallThickness=0.04 % Parameterized on : 09-Jun-2026 19:35:13 m  wallMaterialDen=650 % Parameterized on : 09-Jun-2026 19:35:15 kg/m^3  wallMaterialCp=1100 % Parameterized on : 09-Jun-2026 19:35:15 J/(K*kg)  wallAbsorptivity=0.5  wallThermalK=1.4 % Parameterized on : 09-Jun-2026 19:35:15 W/(K*m)  winLength=1 m  winHeight=0.5 m  winThickness=0.007 m  winMaterialDen=2500 kg/m^3  winMaterialCp=787 J/(K*kg)  winAbsorptivity=0.35  winThermalK=1 W/(K*m)  winTransmissivity=0.45  ventLength=0.1 m  ventHeight=0.1 m  extToWallHTC=30 % Parameterized on : 09-Jun-2026 19:35:15 W/(K*m^2)  intToRoomHTC=30 % Parameterized on : 09-Jun-2026 19:35:15 W/(K*m^2)  iniT=275.8 % Parameterized on : 09-Jun-2026 19:38:28 K
  W_A1R1_A1R5 : WallSelector_lib/Wall Selector  optWall=wallModelOption.wallWinVent  wallLength=0.60966 % Parameterized on : 09-Jun-2026 19:35:13 m  wallHeight=3.048 % Parameterized on : 09-Jun-2026 19:35:13 m  wallThickness=0.04 % Parameterized on : 09-Jun-2026 19:35:13 m  wallMaterialDen=650 % Parameterized on : 09-Jun-2026 19:35:15 kg/m^3  wallMaterialCp=1100 % Parameterized on : 09-Jun-2026 19:35:15 J/(K*kg)  wallAbsorptivity=0.5  wallThermalK=1.4 % Parameterized on : 09-Jun-2026 19:35:15 W/(K*m)  winLength=1 m  winHeight=0.5 m  winThickness=0.007 m  winMaterialDen=2500 kg/m^3  winMaterialCp=787 J/(K*kg)  winAbsorptivity=0.35  winThermalK=1 W/(K*m)  winTransmissivity=0.45  ventLength=0.4311 % Parameterized on : 09-Jun-2026 19:35:13 m  ventHeight=2.1553 % Parameterized on : 09-Jun-2026 19:35:13 m  extToWallHTC=30 % Parameterized on : 09-Jun-2026 19:35:15 W/(K*m^2)  intToRoomHTC=30 % Parameterized on : 09-Jun-2026 19:35:15 W/(K*m^2)  iniT=275.8 % Parameterized on : 09-Jun-2026 19:38:28 K
  W_A1R2_A1R3 : WallSelector_lib/Wall Selector  optWall=wallModelOption.wallOnly  wallLength=0.61001 % Parameterized on : 09-Jun-2026 19:35:13 m  wallHeight=3.048 % Parameterized on : 09-Jun-2026 19:35:13 m  wallThickness=0.04 % Parameterized on : 09-Jun-2026 19:35:13 m  wallMaterialDen=650 % Parameterized on : 09-Jun-2026 19:35:15 kg/m^3  wallMaterialCp=1100 % Parameterized on : 09-Jun-2026 19:35:15 J/(K*kg)  wallAbsorptivity=0.5  wallThermalK=1.4 % Parameterized on : 09-Jun-2026 19:35:15 W/(K*m)  winLength=1 m  winHeight=0.5 m  winThickness=0.007 m  winMaterialDen=2500 kg/m^3  winMaterialCp=787 J/(K*kg)  winAbsorptivity=0.35  winThermalK=1 W/(K*m)  winTransmissivity=0.45  ventLength=0.1 m  ventHeight=0.1 m  extToWallHTC=30 % Parameterized on : 09-Jun-2026 19:35:15 W/(K*m^2)  intToRoomHTC=30 % Parameterized on : 09-Jun-2026 19:35:15 W/(K*m^2)  iniT=275.8 % Parameterized on : 09-Jun-2026 19:38:28 K
  W_A1R2_A1R4 : WallSelector_lib/Wall Selector  optWall=wallModelOption.wallWinVent  wallLength=1.2188 % Parameterized on : 09-Jun-2026 19:35:13 m  wallHeight=3.048 % Parameterized on : 09-Jun-2026 19:35:13 m  wallThickness=0.04 % Parameterized on : 09-Jun-2026 19:35:13 m  wallMaterialDen=650 % Parameterized on : 09-Jun-2026 19:35:15 kg/m^3  wallMaterialCp=1100 % Parameterized on : 09-Jun-2026 19:35:15 J/(K*kg)  wallAbsorptivity=0.5  wallThermalK=1.4 % Parameterized on : 09-Jun-2026 19:35:15 W/(K*m)  winLength=1 m  winHeight=0.5 m  winThickness=0.007 m  winMaterialDen=2500 kg/m^3  winMaterialCp=787 J/(K*kg)  winAbsorptivity=0.35  winThermalK=1 W/(K*m)  winTransmissivity=0.45  ventLength=0.60942 % Parameterized on : 09-Jun-2026 19:35:13 m  ventHeight=1.524 % Parameterized on : 09-Jun-2026 19:35:13 m  extToWallHTC=30 % Parameterized on : 09-Jun-2026 19:35:15 W/(K*m^2)  intToRoomHTC=30 % Parameterized on : 09-Jun-2026 19:35:15 W/(K*m^2)  iniT=275.8 % Parameterized on : 09-Jun-2026 19:38:28 K
  W_A1R3_A1R5 : WallSelector_lib/Wall Selector  optWall=wallModelOption.wallOnly  wallLength=1.5239 % Parameterized on : 09-Jun-2026 19:35:13 m  wallHeight=3.048 % Parameterized on : 09-Jun-2026 19:35:13 m  wallThickness=0.04 % Parameterized on : 09-Jun-2026 19:35:13 m  wallMaterialDen=650 % Parameterized on : 09-Jun-2026 19:35:15 kg/m^3  wallMaterialCp=1100 % Parameterized on : 09-Jun-2026 19:35:15 J/(K*kg)  wallAbsorptivity=0.5  wallThermalK=1.4 % Parameterized on : 09-Jun-2026 19:35:15 W/(K*m)  winLength=1 m  winHeight=0.5 m  winThickness=0.007 m  winMaterialDen=2500 kg/m^3  winMaterialCp=787 J/(K*kg)  winAbsorptivity=0.35  winThermalK=1 W/(K*m)  winTransmissivity=0.45  ventLength=0.1 m  ventHeight=0.1 m  extToWallHTC=30 % Parameterized on : 09-Jun-2026 19:35:15 W/(K*m^2)  intToRoomHTC=30 % Parameterized on : 09-Jun-2026 19:35:15 W/(K*m^2)  iniT=275.8 % Parameterized on : 09-Jun-2026 19:38:28 K
  roomT : Subsystem
  Amb : PMIOPort  Side=Left
  Solar : PMIOPort  Port=2  Side=Left
  S : PMIOPort  Port=3  Side=Left
  Top : PMIOPort  Port=4  Side=Left
  T : PMIOPort  Port=5  Side=Right
  Bottom : PMIOPort  Port=6  Side=Right
  connections:
  Room_A1R1_LivingRoom/RConn1 -- W_A1R1_A1R2/RConn1
  W_A1R1_A1R2/LConn1 -- Room_A1R2_Bedroom/LConn2 -- W_A1R2_A1R3/RConn1 -- W_A1R2_A1R4/RConn1
  W_A1R1_A1R3/RConn1 -- Room_A1R1_LivingRoom/LConn3 -- W_A1R1_A1R5/RConn1
  Room_A1R3_Kitchen/RConn3 -- W_A1R1_A1R3/LConn1
  W_A1R1_A1R4/RConn1 -- Room_A1R1_LivingRoom/RConn3 -- ExtWall (A1R1W2)/RConn1
  Room_A1R4_Bathroom/LConn3 -- W_A1R1_A1R4/LConn1
  W_A1R1_A1R5/LConn1 -- Room_A1R5_FireExit/RConn3 -- ExtWall (A1R5W2)/RConn1
  W_A1R2_A1R3/LConn1 -- Room_A1R3_Kitchen/RConn1 -- ExtWall (A1R3W3)/RConn1
  W_A1R2_A1R4/LConn1 -- Room_A1R4_Bathroom/RConn1 -- ExtWall (A1R4W3)/RConn1
  W_A1R3_A1R5/RConn1 -- Room_A1R3_Kitchen/LConn2 -- ExtWall (A1R3W1)/RConn1
  Room_A1R5_FireExit/RConn1 -- W_A1R3_A1R5/LConn1
  Room_A1R1_LivingRoom/LConn2 -- ExtWall (A1R1W1)/RConn1
  ExtWall (A1R1W1)/LConn2 -- Amb1/LConn1
  ExtWall (A1R1W2)/LConn2 -- Amb2/LConn1
  Room_A1R2_Bedroom/RConn3 -- ExtWall (A1R2W2)/RConn1
  ExtWall (A1R2W2)/LConn2 -- Amb3/LConn1
  Room_A1R2_Bedroom/RConn1 -- ExtWall (A1R2W3)/RConn1
  ExtWall (A1R2W3)/LConn2 -- Amb4/LConn1
  Room_A1R2_Bedroom/LConn3 -- ExtWall (A1R2W4)/RConn1
  ExtWall (A1R2W4)/LConn2 -- Amb5/LConn1
  ExtWall (A1R3W1)/LConn2 -- Amb6/LConn1
  ExtWall (A1R3W3)/LConn2 -- Amb7/LConn1
  Room_A1R3_Kitchen/LConn3 -- ExtWall (A1R3W4)/RConn1
  ExtWall (A1R3W4)/LConn2 -- Amb8/LConn1
  Room_A1R4_Bathroom/LConn2 -- ExtWall (A1R4W1)/RConn1
  ExtWall (A1R4W1)/LConn2 -- Amb9/LConn1
  Room_A1R4_Bathroom/RConn3 -- ExtWall (A1R4W2)/RConn1
  ExtWall (A1R4W2)/LConn2 -- Amb10/LConn1
  ExtWall (A1R4W3)/LConn2 -- Amb11/LConn1
  Room_A1R5_FireExit/LConn2 -- ExtWall (A1R5W1)/RConn1
  ExtWall (A1R5W1)/LConn2 -- Amb12/LConn1
  ExtWall (A1R5W2)/LConn2 -- Amb13/LConn1
  Room_A1R5_FireExit/LConn3 -- ExtWall (A1R5W4)/RConn1
  ExtWall (A1R5W4)/LConn2 -- Amb14/LConn1
  Amb/RConn1 -- AmbPort/LConn1
  ExtWall (A1R1W1)/LConn1 -- ExtWall (A1R1W2)/LConn1 -- ExtWall (A1R2W2)/LConn1 -- ExtWall (A1R2W3)/LConn1 -- ExtWall (A1R2W4)/LConn1 -- ExtWall (A1R3W1)/LConn1 -- ExtWall (A1R3W3)/LConn1 -- ExtWall (A1R3W4)/LConn1 -- ExtWall (A1R4W1)/LConn1 -- ExtWall (A1R4W2)/LConn1 -- ExtWall (A1R4W3)/LConn1 -- ExtWall (A1R5W1)/LConn1 -- ExtWall (A1R5W2)/LConn1 -- Solar/RConn1 -- ExtWall (A1R5W4)/LConn1
  roomT/LConn1 -- Room_A1R1_LivingRoom/RConn2
  roomT/LConn2 -- Room_A1R2_Bedroom/RConn2
  roomT/LConn3 -- Room_A1R3_Kitchen/RConn2
  roomT/LConn4 -- Room_A1R4_Bathroom/RConn2
  roomT/LConn5 -- Room_A1R5_FireExit/RConn2
  roomT/RConn1 -- T/RConn1
  Room_A1R1_LivingRoom/LConn1 -- Room_A1R2_Bedroom/LConn1 -- Room_A1R3_Kitchen/LConn1 -- Room_A1R4_Bathroom/LConn1 -- S/RConn1 -- Room_A1R5_FireExit/LConn1
  Top1/LConn1 -- ArrayTop/LConn1
  Top2/LConn1 -- ArrayTop/LConn2
  Top3/LConn1 -- ArrayTop/LConn3
  Top4/LConn1 -- ArrayTop/LConn4
  Top5/LConn1 -- ArrayTop/LConn5
  ArrayTop/RConn1 -- Top/RConn1
  Room_A1R1_LivingRoom/LConn4 -- Top1Lib/LConn1
  Room_A1R2_Bedroom/LConn4 -- Top2Lib/LConn1
  Room_A1R3_Kitchen/LConn4 -- Top3Lib/LConn1
  Room_A1R4_Bathroom/LConn4 -- Top4Lib/LConn1
  Room_A1R5_FireExit/LConn4 -- Top5Lib/LConn1
  Bottom1/LConn1 -- ArrayBottom/LConn1
  Bottom2/LConn1 -- ArrayBottom/LConn2
  Bottom3/LConn1 -- ArrayBottom/LConn3
  Bottom4/LConn1 -- ArrayBottom/LConn4
  Bottom5/LConn1 -- ArrayBottom/LConn5
  ArrayBottom/RConn1 -- Bottom/RConn1
  Room_A1R1_LivingRoom/RConn4 -- Bottom1Lib/LConn1
  Room_A1R2_Bedroom/RConn4 -- Bottom2Lib/LConn1
  Room_A1R3_Kitchen/RConn4 -- Bottom3Lib/LConn1
  Room_A1R4_Bathroom/RConn4 -- Bottom4Lib/LConn1
  Room_A1R5_FireExit/RConn4 -- Bottom5Lib/LConn1
